simulink model "AutoRS_Antriebsstrang_Simulink"  (R2022b)
settings: Solver=FixedStepAuto  StartTime=0.0  StopTime=50  FixedStep=1e-4  RelTol=1e-3
undefined symbols (not defined in the file): M_g_final, M_r_final, param_const
settings Model: Creator=Sebastian  LastModifiedBy=Aaron

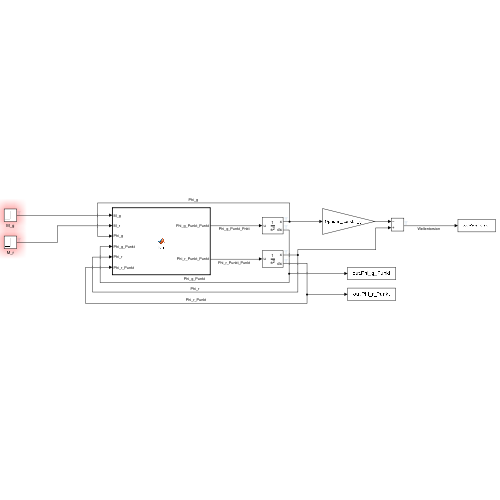
[thumbnail: Simulink's stored preview of the top-level diagram]
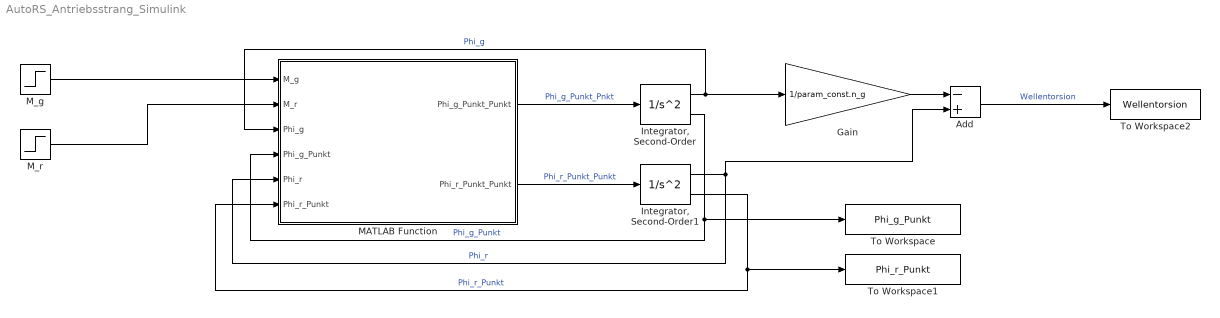
== system AutoRS_Antriebsstrang_Simulink ==
  Add : Sum  Inputs=-+
  Gain : Gain  Gain=1/param_const.n_g
  "Integrator, Second-Order" : SecondOrderIntegrator
  "Integrator, Second-Order1" : SecondOrderIntegrator
  MATLAB Function : MATLAB Function  TreatAsAtomicUnit=on
  M_g : Step  Time=15  After=M_g_final  SampleTime=0
  M_r : Step  Time=5  After=M_r_final  SampleTime=0
  To Workspace : ToWorkspace  VariableName=Phi_g_Punkt  SaveFormat=Timeseries  SampleTime=-1
  To Workspace1 : ToWorkspace  VariableName=Phi_r_Punkt  SaveFormat=Timeseries  SampleTime=-1
  To Workspace2 : ToWorkspace  VariableName=Wellentorsion  SaveFormat=Timeseries  SampleTime=-1
  wires:
  MATLAB Function/2(Phi_r_Punkt_Punkt) -> "Integrator, Second-Order1"/1  "Phi_r_Punkt_Punkt"
  MATLAB Function/1(Phi_g_Punkt_Punkt) -> "Integrator, Second-Order"/1  "Phi_g_Punkt_Pnkt"
  "Integrator, Second-Order"/2 -> MATLAB Function/4(Phi_g_Punkt), To Workspace/1  "Phi_g_Punkt"
  "Integrator, Second-Order"/1 -> Gain/1, MATLAB Function/3(Phi_g)  "Phi_g"
  "Integrator, Second-Order1"/2 -> MATLAB Function/6(Phi_r_Punkt), To Workspace1/1  "Phi_r_Punkt"
  "Integrator, Second-Order1"/1 -> Add/2, MATLAB Function/5(Phi_r)  "Phi_r"
  M_g/1 -> MATLAB Function/1(M_g)
  M_r/1 -> MATLAB Function/2(M_r)
  Gain/1 -> Add/1
  Add/1 -> To Workspace2/1  "Wellentorsion"

== matlab function AutoRS_Antriebsstrang_Simulink/MATLAB Function ==
  data: M_g input; M_r input; Phi_g_Punkt_Punkt output; Phi_r_Punkt_Punkt output; Phi_g input; Phi_g_Punkt input; Phi_r input; Phi_r_Punkt input; param_const parameter
function [Phi_g_Punkt_Punkt, Phi_r_Punkt_Punkt]= fcn(M_g, M_r, Phi_g, Phi_g_Punkt, Phi_r, Phi_r_Punkt, param_const)

    Phi_g_Punkt_Punkt = (-param_const.k_s*(Phi_g-param_const.n_g*Phi_r)-param_const.d_s*(Phi_g_Punkt-param_const.n_g*Phi_r_Punkt)-M_g)/param_const.J_g;

    Phi_r_Punkt_Punkt = (M_r-param_const.n_g*(param_const.k_s*(param_const.n_g*Phi_r-Phi_g))-param_const.n_g*(param_const.d_s*(param_const.n_g*Phi_r_Punkt-Phi_g_Punkt)))/param_const.J_r;

end
